simulink model "sinewave"  (R2024b)
settings: Solver=VariableStepAuto  StartTime=0.0  StopTime=10.0  RelTol=1e-3
settings Model: Creator=sanja  LastModifiedBy=sanja

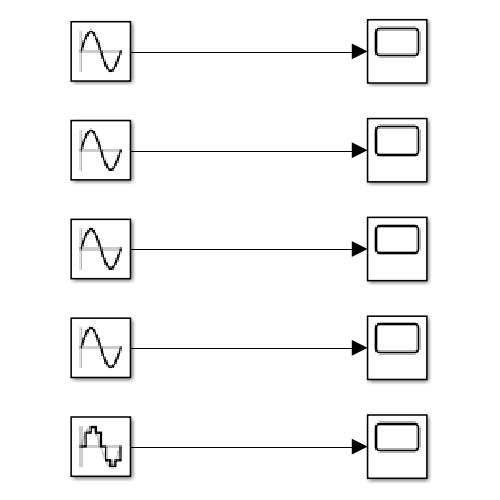
[thumbnail: Simulink's stored preview of the top-level diagram]
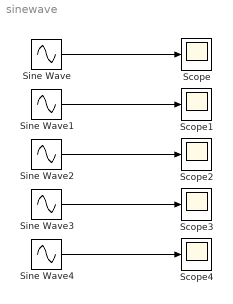
== system sinewave ==
  Scope{,1..4} (5 alike) : Scope
  Sine Wave : Sin  Bias=5  SampleTime=0
  Sine Wave1 : Sin  Amplitude=70*sqrt(2)  SampleTime=0
  Sine Wave2 : Sin  Frequency=50*2*pi  SampleTime=0
  Sine Wave3 : Sin  Phase=2  SampleTime=0
  Sine Wave4 : Sin  SampleTime=0.2
  wires:
  Sine Wave/1 -> Scope/1
  Sine Wave1/1 -> Scope1/1
  Sine Wave2/1 -> Scope2/1
  Sine Wave3/1 -> Scope3/1
  Sine Wave4/1 -> Scope4/1
